simulink model "ruido"  (Simulink 5.0)
settings: Solver=ode45  StartTime=0.0  StopTime=10.0  RelTol=1e-3
settings Model: LastModifiedBy=Invitado

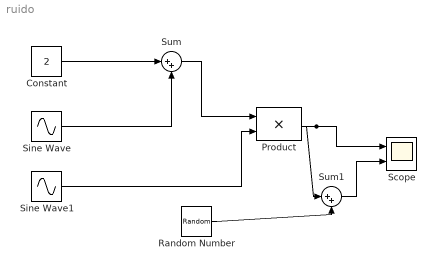
== system ruido ==
  Constant : Constant  Value=2
  Product : Product  SaturateOnIntegerOverflow=on
  Random Number : RandomNumber  SampleTime=0
  Scope : Scope  NumInputPorts=2
      settings: TimeRange=10  YMin=-5~-5  YMax=5~5  SampleTime=0.01
  Sine Wave : Sin  Amplitude=2  SampleTime=0.01
  Sine Wave1 : Sin  Amplitude=2  Frequency=20  SampleTime=0.01
  Sum : Sum  Inputs=|++  SaturateOnIntegerOverflow=on
  Sum1 : Sum  Inputs=|++  SaturateOnIntegerOverflow=on
  wires:
  Constant/1 -> Sum/1
  Sine Wave/1 -> Sum/2
  Sum/1 -> Product/1
  Sine Wave1/1 -> Product/2
  Random Number/1 -> Sum1/2
  Product/1 -> Scope/1, Sum1/1
  Sum1/1 -> Scope/2
